simulink model "Plant_linearized"  (R2023a)
settings: Solver=VariableStepAuto  StartTime=0.0  StopTime=10102  RelTol=1e-3
values from neighbouring files (symbols this model uses):
  A = Plant_completo_orig_mod_Timed_Based_Linearization_nominal.a    [BodeAnalysis.m]    (also in colonna2.m = [1+xa(i)*aalfa(1)/xs xa(i)*aalfa(1)/xs xa(i)*aalfa(1)/xs;   ; create_csv_completo_linearized.m = Timed_Based_Linearization_nominal_1e50.a)
  B = Plant_completo_orig_mod_Timed_Based_Linearization_nominal.b    [BodeAnalysis.m]    (also in colonna2.m = [aalfa(1)*xa(i)/xs;aalfa(2)*xb(i)/xs;aalfa(3)*xc(i)/xs]; create_csv_completo_linearized.m = Timed_Based_Linearization_nominal_1e50.b)
  C = Plant_completo_orig_mod_Timed_Based_Linearization_nominal.c    [BodeAnalysis.m]    (also in create_csv_completo_linearized.m = Timed_Based_Linearization_nominal_1e50.c)
  D = Plant_completo_orig_mod_Timed_Based_Linearization_nominal.d    [BodeAnalysis.m]    (also in create_csv_completo_linearized.m = Timed_Based_Linearization_nominal_1e50.d)
  F0A = 100    [ChemBenchData.m]    (also in dati.m)
  R1 = 330    [ChemBenchData.m]    (also in dati.m = 400)
  R2 = 283    [ChemBenchData.m]    (also in dati.m = 375)
  R3 = 141    [ChemBenchData.m]    (also in dati.m = 272)
  y_eq = y_eq    [BodeAnalysis.m]    (also in create_csv_completo_linearized.m)
libraries: slident x4
settings Model: Creator=laura  LastModifiedBy=laura

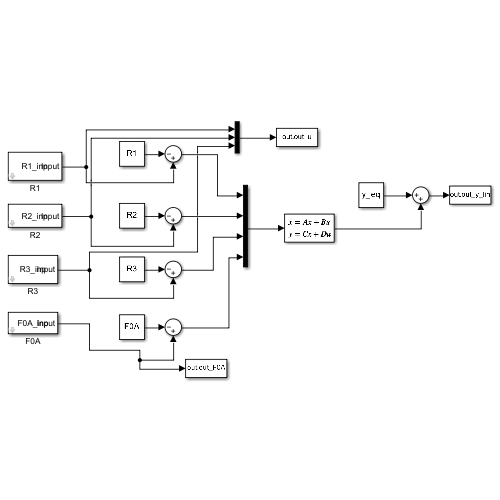
[thumbnail: Simulink's stored preview of the top-level diagram]
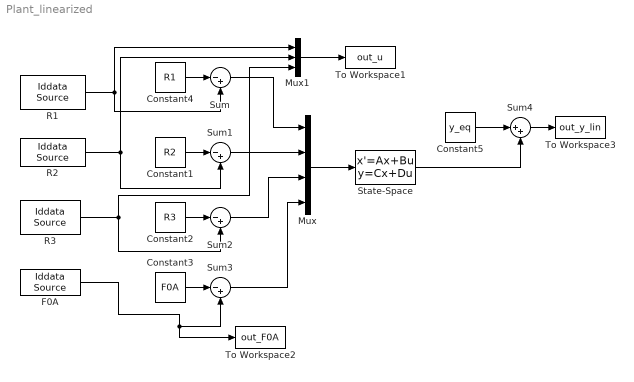
== system Plant_linearized ==
  Constant1 : Constant  Value=R2
  Constant2 : Constant  Value=R3
  Constant3 : Constant  Value=F0A
  Constant4 : Constant  Value=R1
  Constant5 : Constant  Value=y_eq
  F0A : slident/Iddata Source  iddataobj=F0A_inp
  Mux : Mux
  Mux1 : Mux  Inputs=3
  R1 : slident/Iddata Source  iddataobj=R1_inp
  R2 : slident/Iddata Source  iddataobj=R2_inp
  R3 : slident/Iddata Source  iddataobj=R3_inp
  State-Space : StateSpace  A=A  B=B  C=C  D=D  InitialCondition=0
  Sum{,1..3} (4 alike) : Sum  Inputs=|-+
  Sum4 : Sum  Inputs=|++
  To Workspace1 : ToWorkspace  VariableName=out_u  SampleTime=1
  To Workspace2 : ToWorkspace  VariableName=out_F0A  SampleTime=1
  To Workspace3 : ToWorkspace  VariableName=out_y_lin  SampleTime=1
  wires:
  Mux/1 -> State-Space/1
  R1/1 -> Sum/2, Mux1/1
  Constant4/1 -> Sum/1
  Sum/1 -> Mux/1
  Constant1/1 -> Sum1/1
  Sum1/1 -> Mux/2
  R2/1 -> Mux1/2, Sum1/2
  Sum2/1 -> Mux/3
  Constant2/1 -> Sum2/1
  R3/1 -> Mux1/3, Sum2/2
  Constant3/1 -> Sum3/1
  F0A/1 -> To Workspace2/1, Sum3/2
  Sum3/1 -> Mux/4
  Mux1/1 -> To Workspace1/1
  Constant5/1 -> Sum4/1
  State-Space/1 -> Sum4/2
  Sum4/1 -> To Workspace3/1
